simulink model "a_CurrentController_IdealPWMVariousVbusFsw"  (R2013b)
settings: Solver=ode3  StartTime=0.0  StopTime=3e-3  FixedStep=.5e-7  MaxStep=1e-6  RelTol=1e-3
values from neighbouring files (symbols this model uses):
  Ki = R/L*Kp    (= 10000)    [CurrentControllerDesign.m]
  Kp = L*wci    (= 45.2)    [CurrentControllerDesign.m]
  L = 45.2e-3    (= 0.0452)    [CurrentControllerDesign.m]
  R = 10    [CurrentControllerDesign.m]
libraries: fl_lib x28, nesl_utility x14, simulink x6
settings Model: Creator=Eric  LastModifiedBy=sever212
settings DebuggingCC: StateNameClashWarn=warning

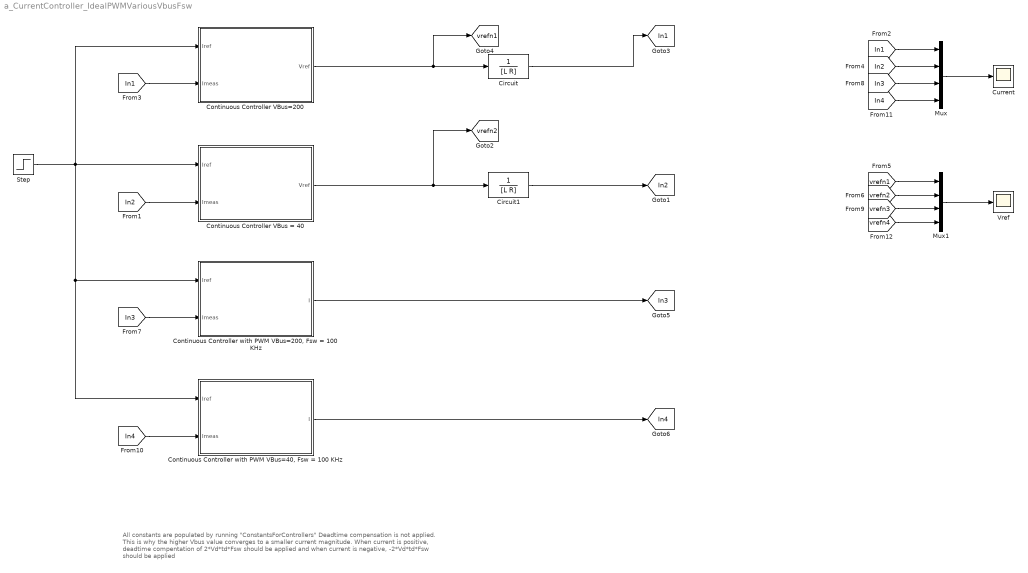
== system a_CurrentController_IdealPWMVariousVbusFsw ==
  note: All constants are populated by running "ConstantsForControllers"
      |
      | Deadtime compensation is not applied. This is why the higher Vbus value converges to a smaller current magnitude.
      |
      | When current is positive, deadtime compentation of 2*Vd*td*Fsw should be applied
      | and when current is negative, -2*Vd*td*Fsw should be applied
  Circuit : TransferFcn  Denominator=[L R]
  Circuit1 : TransferFcn  Denominator=[L R]
  Continuous Controller VBus = 40 : Subsystem  mask{Vdcbus=40}
      mask prompts: Vdcbus "Vdc"
  Continuous Controller VBus=200 : Subsystem  mask{Vdcbus=200}
      mask prompts: Vdcbus "Vdc"
  "Continuous Controller with PWM VBus=200, Fsw = 100 KHz" : Subsystem  mask{Vdcbus=200, fsw=100e3, tdead=80e-9}
      mask prompts: Vdcbus "Vdc"; fsw "Switching Frequency"; tdead "Dead time"
  "Continuous Controller with PWM VBus=40, Fsw = 100 KHz" : Subsystem  mask{Vdcbus=40, fsw=100e3, tdead=80e-9}
      mask prompts: Vdcbus "Vdc"; fsw "Switching Frequency"; tdead "Dead time"
  Current : Scope
      settings: YMin=-1.1  YMax=1.1
  Mux : Mux
  Mux1 : Mux
  Step : Step  Time=1.5e-3  Before=1  After=-1  SampleTime=0
  Vref : Scope
      settings: YMin=-40.5  YMax=-35.5
  tag scope: In1=global, In2=global, In3=global, In4=global, vrefn1=global, vrefn2=global
  wires:
  Continuous Controller VBus=200/1(Vref) -> [vrefn1], Circuit/1
  Circuit/1 -> [In1]
  [In1] -> Continuous Controller VBus=200/2(Imeas)
  [In2] -> Continuous Controller VBus = 40/2(Imeas)
  Continuous Controller VBus = 40/1(Vref) -> [vrefn2], Circuit1/1
  Circuit1/1 -> [In2]
  [In1] -> Mux/1
  [In2] -> Mux/2
  Mux/1 -> Current/1
  [vrefn1] -> Mux1/1
  [vrefn2] -> Mux1/2
  Mux1/1 -> Vref/1
  [In3] -> "Continuous Controller with PWM VBus=200, Fsw = 100 KHz"/2(Imeas)
  "Continuous Controller with PWM VBus=200, Fsw = 100 KHz"/1(I) -> [In3]
  [vrefn3] -> Mux1/3
  [In3] -> Mux/3
  Step/1 -> "Continuous Controller with PWM VBus=200, Fsw = 100 KHz"/1(Iref), "Continuous Controller with PWM VBus=40, Fsw = 100 KHz"/1(Iref), Continuous Controller VBus = 40/1(Iref), Continuous Controller VBus=200/1(Iref)
  [In4] -> "Continuous Controller with PWM VBus=40, Fsw = 100 KHz"/2(Imeas)
  "Continuous Controller with PWM VBus=40, Fsw = 100 KHz"/1(I) -> [In4]
  [In4] -> Mux/4
  [vrefn4] -> Mux1/4

== system a_CurrentController_IdealPWMVariousVbusFsw/Continuous Controller VBus = 40 ==
  Iref : Inport
  Imeas : Inport  Port=2
  Get Error : Subsystem
  PI controller : Subsystem
  Vref : Outport
  wires:
  Get Error/1(Error) -> PI controller/1(error)
  Iref/1 -> Get Error/1(Iref)
  Imeas/1 -> Get Error/2(Imeas)
  PI controller/1(Vref) -> Vref/1

== system a_CurrentController_IdealPWMVariousVbusFsw/Continuous Controller VBus=200 ==
  Iref : Inport
  Imeas : Inport  Port=2
  Get Error : Subsystem
  PI controller : Subsystem
  Vref : Outport
  wires:
  Get Error/1(Error) -> PI controller/1(error)
  Iref/1 -> Get Error/1(Iref)
  Imeas/1 -> Get Error/2(Imeas)
  PI controller/1(Vref) -> Vref/1

== system a_CurrentController_IdealPWMVariousVbusFsw/Continuous Controller with PWM VBus=200, Fsw = 100 KHz ==
  Iref : Inport
  Imeas : Inport  Port=2
  Get Error : Subsystem
  Inverter and Winding2 : Subsystem
  PI controller : Subsystem
  Switching Logic : Subsystem
  Terminator : Terminator
  I : Outport
  tag scope: vrefn3=global
  wires:
  Get Error/1(Error) -> PI controller/1(error)
  Iref/1 -> Get Error/1(Iref)
  Imeas/1 -> Get Error/2(Imeas)
  PI controller/1(Vref) -> [vrefn3], Switching Logic/1(Vref)
  Switching Logic/1(q) -> Inverter and Winding2/1(q)
  Inverter and Winding2/2(V) -> Terminator/1
  Inverter and Winding2/1(I) -> I/1

== system a_CurrentController_IdealPWMVariousVbusFsw/Continuous Controller with PWM VBus=40, Fsw = 100 KHz ==
  Iref : Inport
  Imeas : Inport  Port=2
  Get Error : Subsystem
  Inverter and Winding2 : Subsystem
  PI controller : Subsystem
  Switching Logic : Subsystem
  Terminator : Terminator
  I : Outport
  tag scope: vrefn4=global
  wires:
  Get Error/1(Error) -> PI controller/1(error)
  Iref/1 -> Get Error/1(Iref)
  Imeas/1 -> Get Error/2(Imeas)
  PI controller/1(Vref) -> [vrefn4], Switching Logic/1(Vref)
  Switching Logic/1(q) -> Inverter and Winding2/1(q)
  Inverter and Winding2/2(V) -> Terminator/1
  Inverter and Winding2/1(I) -> I/1

== system a_CurrentController_IdealPWMVariousVbusFsw/Continuous Controller VBus = 40/Get Error ==
  Iref : Inport
  Imeas : Inport  Port=2
  Sum : Sum  Inputs=|+-
  Error : Outport
  wires:
  Sum/1 -> Error/1
  Iref/1 -> Sum/1
  Imeas/1 -> Sum/2

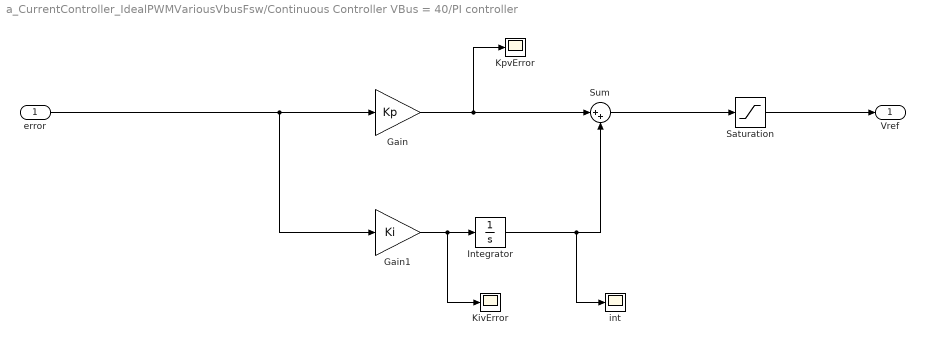
== system a_CurrentController_IdealPWMVariousVbusFsw/Continuous Controller VBus = 40/PI controller ==
  error : Inport
  Gain : Gain  Gain=Kp
  Gain1 : Gain  Gain=Ki
  Integrator : Integrator  LimitOutput=on  UpperSaturationLimit=0.9*Vdcbus  LowerSaturationLimit=-0.9*Vdcbus
  KivError : Scope
      settings: YMin=0.0682  YMax=0.0697  SaveName=ScopeData17
  KpvError : Scope
      settings: YMin=0.0006  YMax=0.00125  SaveName=ScopeData26
  Saturation : Saturate  UpperLimit=0.9*Vdcbus  LowerLimit=-0.9*Vdcbus
  Sum : Sum  Inputs=|++
  int : Scope
      settings: YMin=0.0079765  YMax=0.0079777  SaveName=ScopeData27
  Vref : Outport
  wires:
  error/1 -> Gain1/1, Gain/1
  Gain1/1 -> KivError/1, Integrator/1
  Gain/1 -> KpvError/1, Sum/1
  Integrator/1 -> int/1, Sum/2
  Sum/1 -> Saturation/1
  Saturation/1 -> Vref/1

== system a_CurrentController_IdealPWMVariousVbusFsw/Continuous Controller VBus=200/Get Error ==
  Iref : Inport
  Imeas : Inport  Port=2
  Sum : Sum  Inputs=|+-
  Error : Outport
  wires:
  Sum/1 -> Error/1
  Iref/1 -> Sum/1
  Imeas/1 -> Sum/2

== system a_CurrentController_IdealPWMVariousVbusFsw/Continuous Controller VBus=200/PI controller ==
  error : Inport
  Gain : Gain  Gain=Kp
  Gain1 : Gain  Gain=Ki
  Integrator : Integrator  LimitOutput=on  UpperSaturationLimit=0.9*Vdcbus  LowerSaturationLimit=-0.9*Vdcbus
  KivError : Scope
      settings: YMin=0.0682  YMax=0.0697  SaveName=ScopeData17
  KpvError : Scope
      settings: YMin=0.0006  YMax=0.00125  SaveName=ScopeData26
  Saturation : Saturate  UpperLimit=0.9*Vdcbus  LowerLimit=-0.9*Vdcbus
  Sum : Sum  Inputs=|++
  int : Scope
      settings: YMin=0.0079765  YMax=0.0079777  SaveName=ScopeData27
  Vref : Outport
  wires:
  error/1 -> Gain1/1, Gain/1
  Gain1/1 -> KivError/1, Integrator/1
  Gain/1 -> KpvError/1, Sum/1
  Integrator/1 -> int/1, Sum/2
  Sum/1 -> Saturation/1
  Saturation/1 -> Vref/1

== system a_CurrentController_IdealPWMVariousVbusFsw/Continuous Controller with PWM VBus=200, Fsw = 100 KHz/Get Error ==
  Iref : Inport
  Imeas : Inport  Port=2
  Sum : Sum  Inputs=|+-
  Error : Outport
  wires:
  Sum/1 -> Error/1
  Iref/1 -> Sum/1
  Imeas/1 -> Sum/2

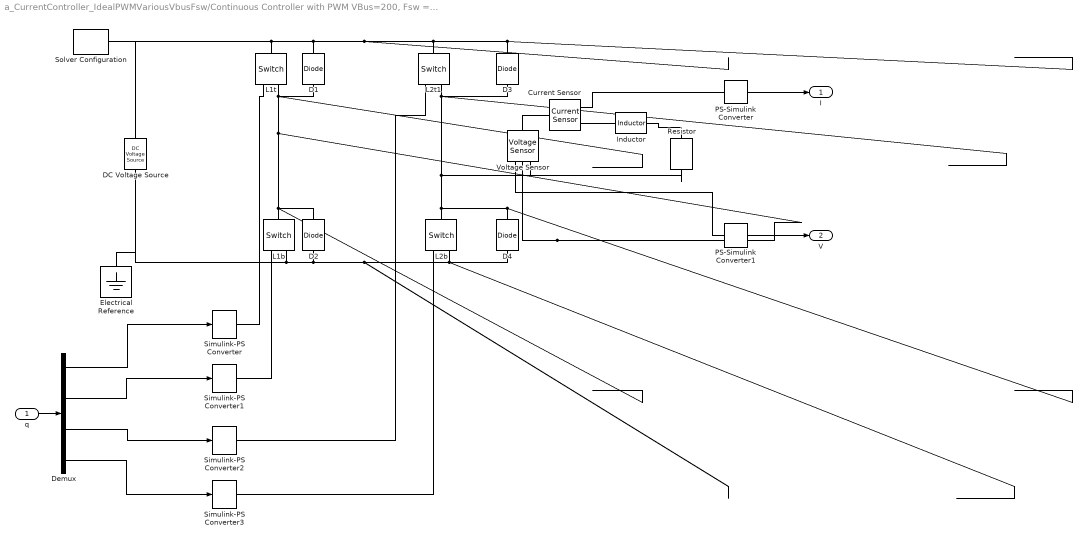
== system a_CurrentController_IdealPWMVariousVbusFsw/Continuous Controller with PWM VBus=200, Fsw = 100 KHz/Inverter and Winding2 ==
  q : Inport
  Current Sensor : fl_lib/Electrical/Electrical Sensors/Current Sensor  i1_Log=off  v1_Log=off  LocalVarNames=|i1|v1  LocalVarDescs=|i1|v1  LocalVarLogging=[0 0]
  D{1..4} (4 alike) : fl_lib/Electrical/Electrical Elements/Diode  Vf=0.15 V  Ron=0.01 Ohm  Goff=1e-7 1/Ohm  i_Log=off  v_Log=off  LocalVarNames=|i|v  LocalVarDescs=|i|v  LocalVarLogging=[0 0]
  DC Voltage Source : fl_lib/Electrical/Electrical Sources/DC Voltage Source  v0=Vdcbus V  i_Log=off  v_Log=off  LocalVarNames=|i|v  LocalVarDescs=|i|v  LocalVarLogging=[0 0]
  Demux : Demux
  Electrical Reference : fl_lib/Electrical/Electrical Elements/Electrical Reference  i_Log=off  LocalVarNames=|i  LocalVarDescs=|i  LocalVarLogging=0
  Inductor : fl_lib/Electrical/Electrical Elements/Inductor  l=L H  i0=0 A  r=0 Ohm  g=1e-8 1/Ohm  i_Log=off  v_Log=off  i_L_Log=off  LocalVarNames=|i|v|i_L  LocalVarDescs=|i|v|Internal variable for current through inductor term  LocalVarLogging=[0 0 0]
  L1b : fl_lib/Electrical/Electrical Elements/Switch  R_closed=0.01 Ohm  G_open=1e-7 1/Ohm  Threshold=0.1  i_Log=off  v_Log=off  LocalVarNames=|i|v  LocalVarDescs=|i|v  LocalVarLogging=[0 0]
  L1t : fl_lib/Electrical/Electrical Elements/Switch  R_closed=0.01 Ohm  G_open=1e-7 1/Ohm  Threshold=0.1  i_Log=off  v_Log=off  LocalVarNames=|i|v  LocalVarDescs=|i|v  LocalVarLogging=[0 0]
  L2b : fl_lib/Electrical/Electrical Elements/Switch  R_closed=0.01 Ohm  G_open=1e-7 1/Ohm  Threshold=0.1  i_Log=off  v_Log=off  LocalVarNames=|i|v  LocalVarDescs=|i|v  LocalVarLogging=[0 0]
  L2t1 : fl_lib/Electrical/Electrical Elements/Switch  R_closed=0.01 Ohm  G_open=1e-7 1/Ohm  Threshold=0.1  i_Log=off  v_Log=off  LocalVarNames=|i|v  LocalVarDescs=|i|v  LocalVarLogging=[0 0]
  PS-Simulink Converter : nesl_utility/PS-Simulink Converter  PhysicalDomain=network_engine_domain  SubClassName=ps_output  LeftPortType=input  RightPortType=output  PseudoPeriodic=off  Frequencies=[]  Unit=1  AffineConversion=off
  PS-Simulink Converter1 : nesl_utility/PS-Simulink Converter  PhysicalDomain=network_engine_domain  SubClassName=ps_output  LeftPortType=input  RightPortType=output  PseudoPeriodic=off  Frequencies=[]  Unit=1  AffineConversion=off
  Resistor : fl_lib/Electrical/Electrical Elements/Resistor  R=R Ohm  i_Log=off  v_Log=off  LocalVarNames=|i|v  LocalVarDescs=|i|v  LocalVarLogging=[0 0]
  Simulink-PS Converter{,1..3} (4 alike) : nesl_utility/Simulink-PS Converter  PhysicalDomain=network_engine_domain  SubClassName=ps_input  LeftPortType=input  RightPortType=output  PseudoPeriodic=off  Frequencies=[]  NoiseDistribution=none  NoiseParameters=[]  Unit=1  AffineConversion=off  InputFiltering=off  SimscapeFilterOrder=1  InputFilterTimeConstant=.001  UdotUserProvided=[]
  Solver Configuration : nesl_utility/Solver Configuration  PhysicalDomain=network_engine_domain  SubClassName=solver  LeftPortType=input  RightPortType=generic  Accelerate=off  Tones=[]  Harmonics=[]  SimulateNoise=off  Profile=off  UseLocalSampling=off  EnableSwitchedLinearOptims=on  FrequencyDomain=off  UseCCode=off  RelTol=0.001  AbsTol=1e-06  MinStep=1e-09  ToWorkspace=off  DoDC=on  ResidualTolerance=1e-8  UseLocalSolver=off  LocalSolverChoice=NE_BACKWARD_EULER_ADVANCER  LocalSolverSampleTime=100e-9  DoFixedCost=off  MaxNonlinIter=15  MaxModeIter=2  LinearAlgebra=Sparse  DelaysMemoryBudget=1024
  Voltage Sensor : fl_lib/Electrical/Electrical Sensors/Voltage Sensor  i1_Log=off  v1_Log=off  LocalVarNames=|i1|v1  LocalVarDescs=|i1|v1  LocalVarLogging=[0 0]
  I : Outport
  V : Outport  Port=2
  wires:
  PS-Simulink Converter/1 -> I/1
  PS-Simulink Converter1/1 -> V/1
  q/1 -> Demux/1
  Demux/1 -> Simulink-PS Converter/1
  Demux/2 -> Simulink-PS Converter1/1
  Demux/3 -> Simulink-PS Converter2/1
  Demux/4 -> Simulink-PS Converter3/1
  connections:
  L1t/RConn2 -- D1/LConn1 -- Voltage Sensor/LConn1 -- Current Sensor/LConn1 -- D2/RConn1 -- L1b/LConn1
  Inductor/RConn1 -- Resistor/LConn1
  Simulink-PS Converter2/RConn1 -- L2t1/RConn1
  Simulink-PS Converter/RConn1 -- L1t/RConn1
  Simulink-PS Converter1/RConn1 -- L1b/RConn1
  D4/RConn1 -- Voltage Sensor/RConn2 -- Resistor/RConn1 -- D3/LConn1 -- L2t1/RConn2 -- L2b/LConn1
  L1b/RConn2 -- Electrical Reference/LConn1 -- DC Voltage Source/RConn1 -- D2/LConn1 -- D4/LConn1 -- L2b/RConn2
  L1t/LConn1 -- L2t1/LConn1 -- D3/RConn1 -- D1/RConn1 -- Solver Configuration/RConn1 -- DC Voltage Source/LConn1
  Simulink-PS Converter3/RConn1 -- L2b/RConn1
  Current Sensor/RConn2 -- Inductor/LConn1
  Current Sensor/RConn1 -- PS-Simulink Converter/LConn1
  Voltage Sensor/RConn1 -- PS-Simulink Converter1/LConn1

== system a_CurrentController_IdealPWMVariousVbusFsw/Continuous Controller with PWM VBus=200, Fsw = 100 KHz/PI controller ==
  error : Inport
  Gain : Gain  Gain=Kp
  Gain1 : Gain  Gain=Ki
  Integrator : Integrator  LimitOutput=on  UpperSaturationLimit=0.9*Vdcbus  LowerSaturationLimit=-0.9*Vdcbus
  KivError : Scope
      settings: YMin=0.0682  YMax=0.0697  SaveName=ScopeData17
  KpvError : Scope
      settings: YMin=0.0006  YMax=0.00125  SaveName=ScopeData26
  Saturation : Saturate  UpperLimit=0.9*Vdcbus  LowerLimit=-0.9*Vdcbus
  Sum : Sum  Inputs=|++
  int : Scope
      settings: YMin=0.0079765  YMax=0.0079777  SaveName=ScopeData27
  Vref : Outport
  wires:
  error/1 -> Gain1/1, Gain/1
  Gain1/1 -> KivError/1, Integrator/1
  Gain/1 -> KpvError/1, Sum/1
  Integrator/1 -> int/1, Sum/2
  Sum/1 -> Saturation/1
  Saturation/1 -> Vref/1

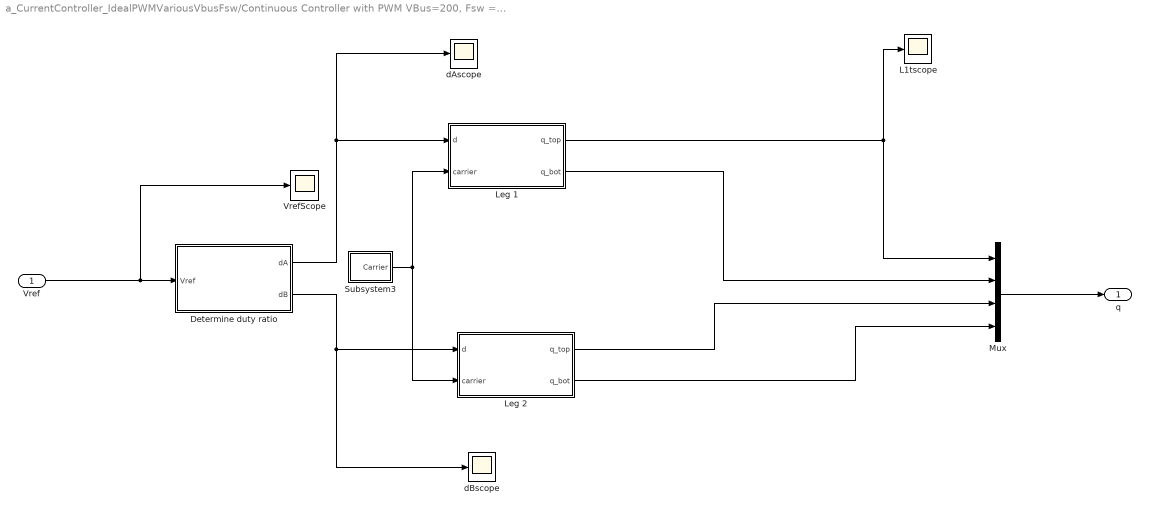
== system a_CurrentController_IdealPWMVariousVbusFsw/Continuous Controller with PWM VBus=200, Fsw = 100 KHz/Switching Logic ==
  Vref : Inport
  Determine duty ratio : Subsystem
  L1tscope : Scope
  Leg 1 : Subsystem
  Leg 2 : Subsystem
  Mux : Mux
  Subsystem3 : Subsystem
  VrefScope : Scope
      settings: YMin=-0.076  YMax=-0.074  SaveName=ScopeData4
  dAscope : Scope
      settings: YMin=0.462  YMax=0.463  SaveName=ScopeData6
  dBscope : Scope
      settings: SaveName=ScopeData7
  q : Outport
  wires:
  Subsystem3/1(Carrier) -> Leg 2/2(carrier), Leg 1/2(carrier)
  Determine duty ratio/2(dB) -> Leg 2/1(d), dBscope/1
  Determine duty ratio/1(dA) -> Leg 1/1(d), dAscope/1
  Vref/1 -> VrefScope/1, Determine duty ratio/1(Vref)
  Leg 1/1(q_top) -> Mux/1, L1tscope/1
  Leg 2/1(q_top) -> Mux/3
  Leg 2/2(q_bot) -> Mux/4
  Mux/1 -> q/1
  Leg 1/2(q_bot) -> Mux/2

== system a_CurrentController_IdealPWMVariousVbusFsw/Continuous Controller with PWM VBus=40, Fsw = 100 KHz/Get Error ==
  Iref : Inport
  Imeas : Inport  Port=2
  Sum : Sum  Inputs=|+-
  Error : Outport
  wires:
  Sum/1 -> Error/1
  Iref/1 -> Sum/1
  Imeas/1 -> Sum/2

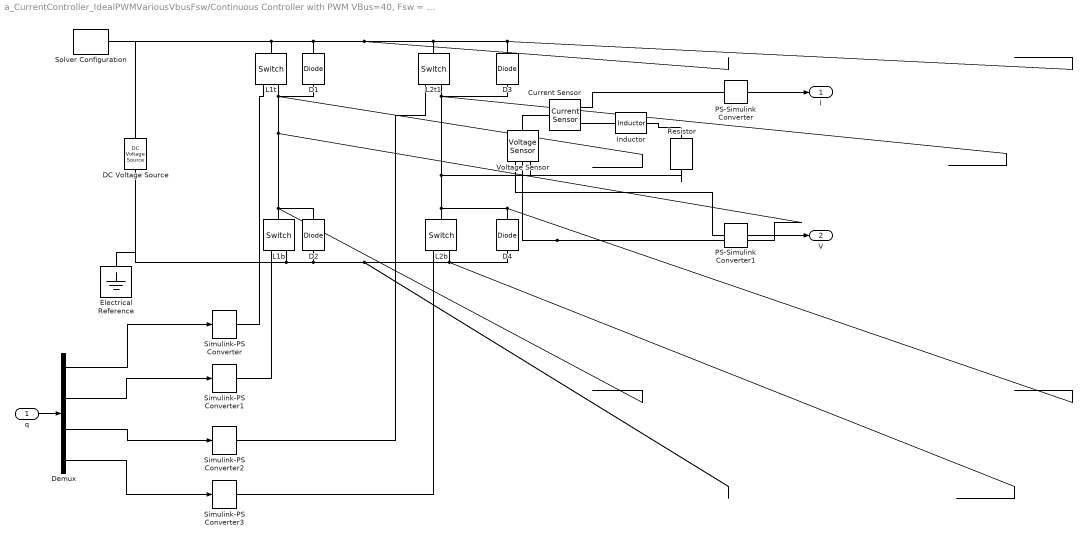
== system a_CurrentController_IdealPWMVariousVbusFsw/Continuous Controller with PWM VBus=40, Fsw = 100 KHz/Inverter and Winding2 ==
  q : Inport
  Current Sensor : fl_lib/Electrical/Electrical Sensors/Current Sensor  i1_Log=off  v1_Log=off  LocalVarNames=|i1|v1  LocalVarDescs=|i1|v1  LocalVarLogging=[0 0]
  D{1..4} (4 alike) : fl_lib/Electrical/Electrical Elements/Diode  Vf=0.15 V  Ron=0.01 Ohm  Goff=1e-7 1/Ohm  i_Log=off  v_Log=off  LocalVarNames=|i|v  LocalVarDescs=|i|v  LocalVarLogging=[0 0]
  DC Voltage Source : fl_lib/Electrical/Electrical Sources/DC Voltage Source  v0=Vdcbus V  i_Log=off  v_Log=off  LocalVarNames=|i|v  LocalVarDescs=|i|v  LocalVarLogging=[0 0]
  Demux : Demux
  Electrical Reference : fl_lib/Electrical/Electrical Elements/Electrical Reference  i_Log=off  LocalVarNames=|i  LocalVarDescs=|i  LocalVarLogging=0
  Inductor : fl_lib/Electrical/Electrical Elements/Inductor  l=L H  i0=0 A  r=0 Ohm  g=1e-8 1/Ohm  i_Log=off  v_Log=off  i_L_Log=off  LocalVarNames=|i|v|i_L  LocalVarDescs=|i|v|Internal variable for current through inductor term  LocalVarLogging=[0 0 0]
  L1b : fl_lib/Electrical/Electrical Elements/Switch  R_closed=0.01 Ohm  G_open=1e-7 1/Ohm  Threshold=0.1  i_Log=off  v_Log=off  LocalVarNames=|i|v  LocalVarDescs=|i|v  LocalVarLogging=[0 0]
  L1t : fl_lib/Electrical/Electrical Elements/Switch  R_closed=0.01 Ohm  G_open=1e-7 1/Ohm  Threshold=0.1  i_Log=off  v_Log=off  LocalVarNames=|i|v  LocalVarDescs=|i|v  LocalVarLogging=[0 0]
  L2b : fl_lib/Electrical/Electrical Elements/Switch  R_closed=0.01 Ohm  G_open=1e-7 1/Ohm  Threshold=0.1  i_Log=off  v_Log=off  LocalVarNames=|i|v  LocalVarDescs=|i|v  LocalVarLogging=[0 0]
  L2t1 : fl_lib/Electrical/Electrical Elements/Switch  R_closed=0.01 Ohm  G_open=1e-7 1/Ohm  Threshold=0.1  i_Log=off  v_Log=off  LocalVarNames=|i|v  LocalVarDescs=|i|v  LocalVarLogging=[0 0]
  PS-Simulink Converter : nesl_utility/PS-Simulink Converter  PhysicalDomain=network_engine_domain  SubClassName=ps_output  LeftPortType=input  RightPortType=output  PseudoPeriodic=off  Frequencies=[]  Unit=1  AffineConversion=off
  PS-Simulink Converter1 : nesl_utility/PS-Simulink Converter  PhysicalDomain=network_engine_domain  SubClassName=ps_output  LeftPortType=input  RightPortType=output  PseudoPeriodic=off  Frequencies=[]  Unit=1  AffineConversion=off
  Resistor : fl_lib/Electrical/Electrical Elements/Resistor  R=R Ohm  i_Log=off  v_Log=off  LocalVarNames=|i|v  LocalVarDescs=|i|v  LocalVarLogging=[0 0]
  Simulink-PS Converter{,1..3} (4 alike) : nesl_utility/Simulink-PS Converter  PhysicalDomain=network_engine_domain  SubClassName=ps_input  LeftPortType=input  RightPortType=output  PseudoPeriodic=off  Frequencies=[]  NoiseDistribution=none  NoiseParameters=[]  Unit=1  AffineConversion=off  InputFiltering=off  SimscapeFilterOrder=1  InputFilterTimeConstant=.001  UdotUserProvided=[]
  Solver Configuration : nesl_utility/Solver Configuration  PhysicalDomain=network_engine_domain  SubClassName=solver  LeftPortType=input  RightPortType=generic  Accelerate=off  Tones=[]  Harmonics=[]  SimulateNoise=off  Profile=off  UseLocalSampling=off  EnableSwitchedLinearOptims=on  FrequencyDomain=off  UseCCode=off  RelTol=0.001  AbsTol=1e-06  MinStep=1e-09  ToWorkspace=off  DoDC=on  ResidualTolerance=1e-8  UseLocalSolver=off  LocalSolverChoice=NE_BACKWARD_EULER_ADVANCER  LocalSolverSampleTime=100e-9  DoFixedCost=off  MaxNonlinIter=15  MaxModeIter=2  LinearAlgebra=Sparse  DelaysMemoryBudget=1024
  Voltage Sensor : fl_lib/Electrical/Electrical Sensors/Voltage Sensor  i1_Log=off  v1_Log=off  LocalVarNames=|i1|v1  LocalVarDescs=|i1|v1  LocalVarLogging=[0 0]
  I : Outport
  V : Outport  Port=2
  wires:
  PS-Simulink Converter/1 -> I/1
  PS-Simulink Converter1/1 -> V/1
  q/1 -> Demux/1
  Demux/1 -> Simulink-PS Converter/1
  Demux/2 -> Simulink-PS Converter1/1
  Demux/3 -> Simulink-PS Converter2/1
  Demux/4 -> Simulink-PS Converter3/1
  connections:
  L1t/RConn2 -- D1/LConn1 -- Voltage Sensor/LConn1 -- Current Sensor/LConn1 -- D2/RConn1 -- L1b/LConn1
  Inductor/RConn1 -- Resistor/LConn1
  Simulink-PS Converter2/RConn1 -- L2t1/RConn1
  Simulink-PS Converter/RConn1 -- L1t/RConn1
  Simulink-PS Converter1/RConn1 -- L1b/RConn1
  D4/RConn1 -- Voltage Sensor/RConn2 -- Resistor/RConn1 -- D3/LConn1 -- L2t1/RConn2 -- L2b/LConn1
  L1b/RConn2 -- Electrical Reference/LConn1 -- DC Voltage Source/RConn1 -- D2/LConn1 -- D4/LConn1 -- L2b/RConn2
  L1t/LConn1 -- L2t1/LConn1 -- D3/RConn1 -- D1/RConn1 -- Solver Configuration/RConn1 -- DC Voltage Source/LConn1
  Simulink-PS Converter3/RConn1 -- L2b/RConn1
  Current Sensor/RConn2 -- Inductor/LConn1
  Current Sensor/RConn1 -- PS-Simulink Converter/LConn1
  Voltage Sensor/RConn1 -- PS-Simulink Converter1/LConn1

== system a_CurrentController_IdealPWMVariousVbusFsw/Continuous Controller with PWM VBus=40, Fsw = 100 KHz/PI controller ==
  error : Inport
  Gain : Gain  Gain=Kp
  Gain1 : Gain  Gain=Ki
  Integrator : Integrator  LimitOutput=on  UpperSaturationLimit=0.9*Vdcbus  LowerSaturationLimit=-0.9*Vdcbus
  KivError : Scope
      settings: YMin=0.0682  YMax=0.0697  SaveName=ScopeData17
  KpvError : Scope
      settings: YMin=0.0006  YMax=0.00125  SaveName=ScopeData26
  Saturation : Saturate  UpperLimit=0.9*Vdcbus  LowerLimit=-0.9*Vdcbus
  Sum : Sum  Inputs=|++
  int : Scope
      settings: YMin=0.0079765  YMax=0.0079777  SaveName=ScopeData27
  Vref : Outport
  wires:
  error/1 -> Gain1/1, Gain/1
  Gain1/1 -> KivError/1, Integrator/1
  Gain/1 -> KpvError/1, Sum/1
  Integrator/1 -> int/1, Sum/2
  Sum/1 -> Saturation/1
  Saturation/1 -> Vref/1

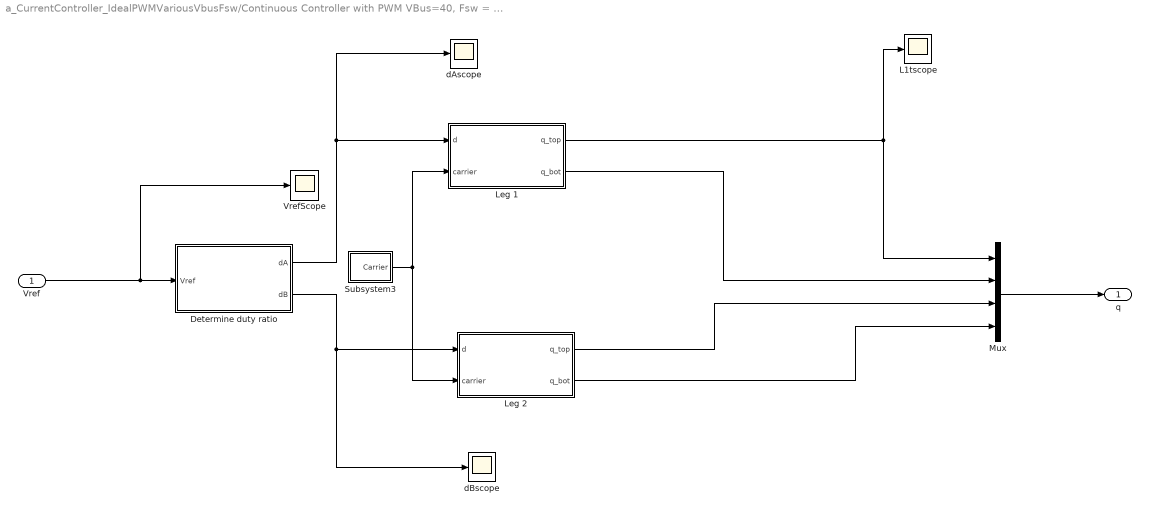
== system a_CurrentController_IdealPWMVariousVbusFsw/Continuous Controller with PWM VBus=40, Fsw = 100 KHz/Switching Logic ==
  Vref : Inport
  Determine duty ratio : Subsystem
  L1tscope : Scope
  Leg 1 : Subsystem
  Leg 2 : Subsystem
  Mux : Mux
  Subsystem3 : Subsystem
  VrefScope : Scope
      settings: YMin=-0.076  YMax=-0.074  SaveName=ScopeData4
  dAscope : Scope
      settings: YMin=0.462  YMax=0.463  SaveName=ScopeData6
  dBscope : Scope
      settings: SaveName=ScopeData7
  q : Outport
  wires:
  Subsystem3/1(Carrier) -> Leg 2/2(carrier), Leg 1/2(carrier)
  Determine duty ratio/2(dB) -> Leg 2/1(d), dBscope/1
  Determine duty ratio/1(dA) -> Leg 1/1(d), dAscope/1
  Vref/1 -> VrefScope/1, Determine duty ratio/1(Vref)
  Leg 1/1(q_top) -> Mux/1, L1tscope/1
  Leg 2/1(q_top) -> Mux/3
  Leg 2/2(q_bot) -> Mux/4
  Mux/1 -> q/1
  Leg 1/2(q_bot) -> Mux/2

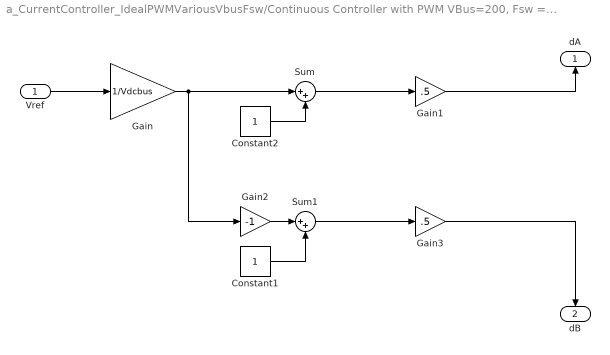
== system a_CurrentController_IdealPWMVariousVbusFsw/Continuous Controller with PWM VBus=200, Fsw = 100 KHz/Switching Logic/Determine duty ratio ==
  Vref : Inport
  Constant1 : Constant
  Constant2 : Constant
  Gain : Gain  Gain=1/Vdcbus
  Gain1 : Gain  Gain=.5
  Gain2 : Gain  Gain=-1
  Gain3 : Gain  Gain=.5
  Sum : Sum  Inputs=|++
  Sum1 : Sum  Inputs=|++
  dA : Outport
  dB : Outport  Port=2
  wires:
  Vref/1 -> Gain/1
  Gain/1 -> Gain2/1, Sum/1
  Sum/1 -> Gain1/1
  Gain2/1 -> Sum1/1
  Gain1/1 -> dA/1
  Constant2/1 -> Sum/2
  Constant1/1 -> Sum1/2
  Sum1/1 -> Gain3/1
  Gain3/1 -> dB/1

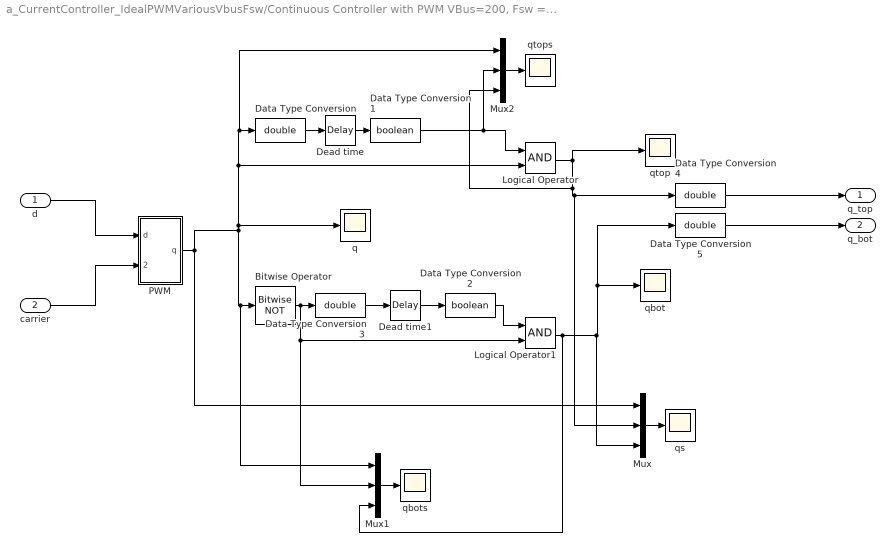
== system a_CurrentController_IdealPWMVariousVbusFsw/Continuous Controller with PWM VBus=200, Fsw = 100 KHz/Switching Logic/Leg 1 ==
  d : Inport
  carrier : Inport  Port=2
  Bitwise Operator : simulink/Logic and Bit Operations/Bitwise Operator  logicop=NOT  UseBitMask=off  BitMask=bin2dec('11011001')  BitMaskRealWorld=Stored Integer
  Data Type Conversion{,3..5} (4 alike) : DataTypeConversion  OutDataTypeStr=double
  Data Type Conversion1 : DataTypeConversion  OutDataTypeStr=boolean
  Data Type Conversion2 : DataTypeConversion  OutDataTypeStr=boolean
  Dead time : TransportDelay  DelayTime=tdead
  Dead time1 : TransportDelay  DelayTime=tdead
  Logical Operator : Logic  AllPortsSameDT=off  OutDataTypeStr=boolean
  Logical Operator1 : Logic  AllPortsSameDT=off  OutDataTypeStr=boolean
  Mux : Mux  Inputs=3
  Mux1 : Mux  Inputs=3
  Mux2 : Mux  Inputs=3
  PWM : Subsystem
  q : Scope
      settings: SaveName=ScopeData5
  qbot : Scope
      settings: SaveName=ScopeData8
  qbots : Scope
      settings: SaveName=ScopeData11
  qs : Scope
      settings: SaveName=ScopeData10
  qtop : Scope
      settings: SaveName=ScopeData9
  qtops : Scope
      settings: YMin=-0.1  YMax=2  SaveName=ScopeData12
  q_top : Outport
  q_bot : Outport  Port=2
  wires:
  d/1 -> PWM/1(d)
  PWM/1(q) -> Mux/1, Mux1/1, Bitwise Operator/1, q/1, Mux2/1, Data Type Conversion/1, Logical Operator/2
  Logical Operator/1 -> Mux2/3, Mux/2, Data Type Conversion4/1, qtop/1
  carrier/1 -> PWM/2(carrier)
  Dead time/1 -> Data Type Conversion1/1
  Bitwise Operator/1 -> Logical Operator1/2, Mux1/2, Data Type Conversion3/1
  Dead time1/1 -> Data Type Conversion2/1
  Logical Operator1/1 -> Mux1/3, Mux/3, qbot/1, Data Type Conversion5/1
  Data Type Conversion1/1 -> Mux2/2, Logical Operator/1
  Data Type Conversion/1 -> Dead time/1
  Data Type Conversion2/1 -> Logical Operator1/1
  Data Type Conversion3/1 -> Dead time1/1
  Mux/1 -> qs/1
  Mux1/1 -> qbots/1
  Mux2/1 -> qtops/1
  Data Type Conversion4/1 -> q_top/1
  Data Type Conversion5/1 -> q_bot/1

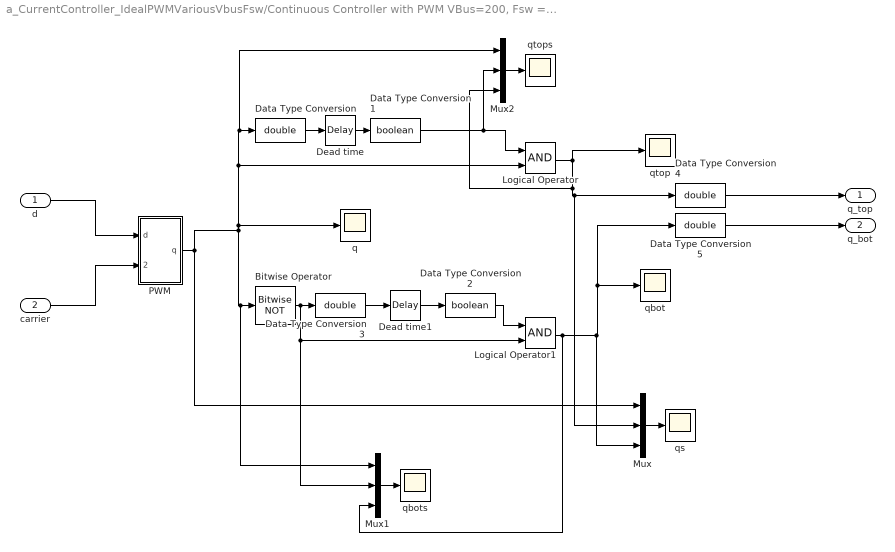
== system a_CurrentController_IdealPWMVariousVbusFsw/Continuous Controller with PWM VBus=200, Fsw = 100 KHz/Switching Logic/Leg 2 ==
  d : Inport
  carrier : Inport  Port=2
  Bitwise Operator : simulink/Logic and Bit Operations/Bitwise Operator  logicop=NOT  UseBitMask=off  BitMask=bin2dec('11011001')  BitMaskRealWorld=Stored Integer
  Data Type Conversion{,3..5} (4 alike) : DataTypeConversion  OutDataTypeStr=double
  Data Type Conversion1 : DataTypeConversion  OutDataTypeStr=boolean
  Data Type Conversion2 : DataTypeConversion  OutDataTypeStr=boolean
  Dead time : TransportDelay  DelayTime=tdead
  Dead time1 : TransportDelay  DelayTime=tdead
  Logical Operator : Logic  AllPortsSameDT=off  OutDataTypeStr=boolean
  Logical Operator1 : Logic  AllPortsSameDT=off  OutDataTypeStr=boolean
  Mux : Mux  Inputs=3
  Mux1 : Mux  Inputs=3
  Mux2 : Mux  Inputs=3
  PWM : Subsystem
  q : Scope
      settings: SaveName=ScopeData5
  qbot : Scope
      settings: SaveName=ScopeData8
  qbots : Scope
      settings: SaveName=ScopeData11
  qs : Scope
      settings: SaveName=ScopeData10
  qtop : Scope
      settings: SaveName=ScopeData9
  qtops : Scope
      settings: YMin=-0.1  YMax=2  SaveName=ScopeData12
  q_top : Outport
  q_bot : Outport  Port=2
  wires:
  d/1 -> PWM/1(d)
  PWM/1(q) -> Mux/1, Mux1/1, Bitwise Operator/1, q/1, Mux2/1, Data Type Conversion/1, Logical Operator/2
  Logical Operator/1 -> Mux2/3, Mux/2, Data Type Conversion4/1, qtop/1
  carrier/1 -> PWM/2(carrier)
  Dead time/1 -> Data Type Conversion1/1
  Bitwise Operator/1 -> Logical Operator1/2, Mux1/2, Data Type Conversion3/1
  Dead time1/1 -> Data Type Conversion2/1
  Logical Operator1/1 -> Mux1/3, Mux/3, qbot/1, Data Type Conversion5/1
  Data Type Conversion1/1 -> Mux2/2, Logical Operator/1
  Data Type Conversion/1 -> Dead time/1
  Data Type Conversion2/1 -> Logical Operator1/1
  Data Type Conversion3/1 -> Dead time1/1
  Mux/1 -> qs/1
  Mux1/1 -> qbots/1
  Mux2/1 -> qtops/1
  Data Type Conversion4/1 -> q_top/1
  Data Type Conversion5/1 -> q_bot/1

== system a_CurrentController_IdealPWMVariousVbusFsw/Continuous Controller with PWM VBus=200, Fsw = 100 KHz/Switching Logic/Subsystem3 ==
  Carrier signal : simulink/Sources/Repeating Sequence  rep_seq_t=[0 .5 1]/fsw  rep_seq_y=[0 1 0]
  Scope : Scope
      settings: SaveName=ScopeData3
  Carrier : Outport
  wires:
  Carrier signal/1 -> Scope/1, Carrier/1

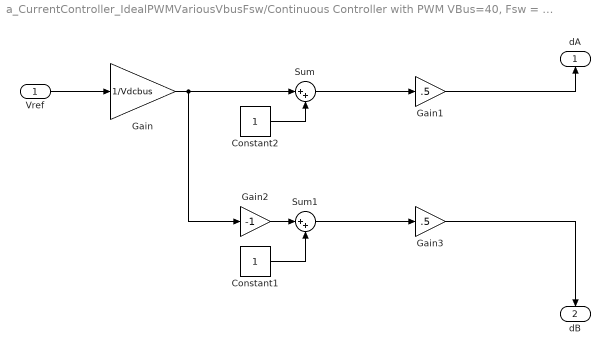
== system a_CurrentController_IdealPWMVariousVbusFsw/Continuous Controller with PWM VBus=40, Fsw = 100 KHz/Switching Logic/Determine duty ratio ==
  Vref : Inport
  Constant1 : Constant
  Constant2 : Constant
  Gain : Gain  Gain=1/Vdcbus
  Gain1 : Gain  Gain=.5
  Gain2 : Gain  Gain=-1
  Gain3 : Gain  Gain=.5
  Sum : Sum  Inputs=|++
  Sum1 : Sum  Inputs=|++
  dA : Outport
  dB : Outport  Port=2
  wires:
  Vref/1 -> Gain/1
  Gain/1 -> Gain2/1, Sum/1
  Sum/1 -> Gain1/1
  Gain2/1 -> Sum1/1
  Gain1/1 -> dA/1
  Constant2/1 -> Sum/2
  Constant1/1 -> Sum1/2
  Sum1/1 -> Gain3/1
  Gain3/1 -> dB/1

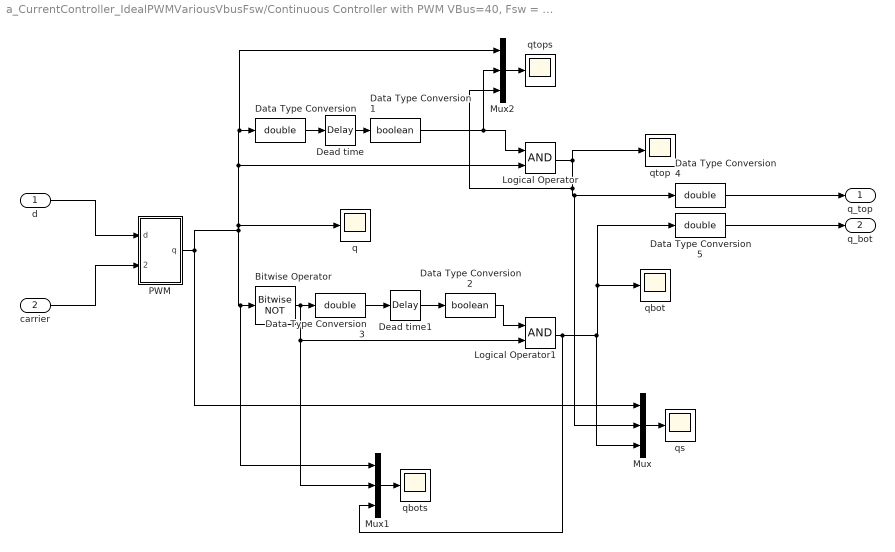
== system a_CurrentController_IdealPWMVariousVbusFsw/Continuous Controller with PWM VBus=40, Fsw = 100 KHz/Switching Logic/Leg 1 ==
  d : Inport
  carrier : Inport  Port=2
  Bitwise Operator : simulink/Logic and Bit Operations/Bitwise Operator  logicop=NOT  UseBitMask=off  BitMask=bin2dec('11011001')  BitMaskRealWorld=Stored Integer
  Data Type Conversion{,3..5} (4 alike) : DataTypeConversion  OutDataTypeStr=double
  Data Type Conversion1 : DataTypeConversion  OutDataTypeStr=boolean
  Data Type Conversion2 : DataTypeConversion  OutDataTypeStr=boolean
  Dead time : TransportDelay  DelayTime=tdead
  Dead time1 : TransportDelay  DelayTime=tdead
  Logical Operator : Logic  AllPortsSameDT=off  OutDataTypeStr=boolean
  Logical Operator1 : Logic  AllPortsSameDT=off  OutDataTypeStr=boolean
  Mux : Mux  Inputs=3
  Mux1 : Mux  Inputs=3
  Mux2 : Mux  Inputs=3
  PWM : Subsystem
  q : Scope
      settings: SaveName=ScopeData5
  qbot : Scope
      settings: SaveName=ScopeData8
  qbots : Scope
      settings: SaveName=ScopeData11
  qs : Scope
      settings: SaveName=ScopeData10
  qtop : Scope
      settings: SaveName=ScopeData9
  qtops : Scope
      settings: YMin=-0.1  YMax=2  SaveName=ScopeData12
  q_top : Outport
  q_bot : Outport  Port=2
  wires:
  d/1 -> PWM/1(d)
  PWM/1(q) -> Mux/1, Mux1/1, Bitwise Operator/1, q/1, Mux2/1, Data Type Conversion/1, Logical Operator/2
  Logical Operator/1 -> Mux2/3, Mux/2, Data Type Conversion4/1, qtop/1
  carrier/1 -> PWM/2(carrier)
  Dead time/1 -> Data Type Conversion1/1
  Bitwise Operator/1 -> Logical Operator1/2, Mux1/2, Data Type Conversion3/1
  Dead time1/1 -> Data Type Conversion2/1
  Logical Operator1/1 -> Mux1/3, Mux/3, qbot/1, Data Type Conversion5/1
  Data Type Conversion1/1 -> Mux2/2, Logical Operator/1
  Data Type Conversion/1 -> Dead time/1
  Data Type Conversion2/1 -> Logical Operator1/1
  Data Type Conversion3/1 -> Dead time1/1
  Mux/1 -> qs/1
  Mux1/1 -> qbots/1
  Mux2/1 -> qtops/1
  Data Type Conversion4/1 -> q_top/1
  Data Type Conversion5/1 -> q_bot/1

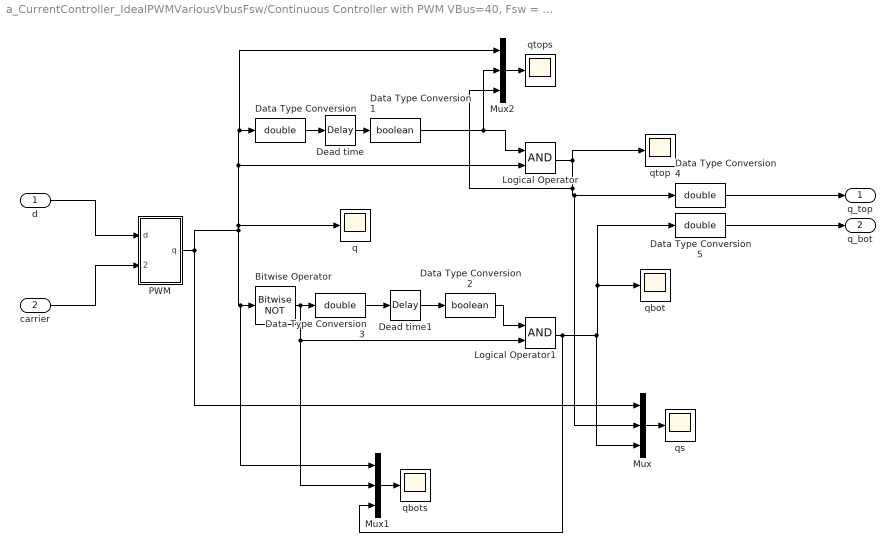
== system a_CurrentController_IdealPWMVariousVbusFsw/Continuous Controller with PWM VBus=40, Fsw = 100 KHz/Switching Logic/Leg 2 ==
  d : Inport
  carrier : Inport  Port=2
  Bitwise Operator : simulink/Logic and Bit Operations/Bitwise Operator  logicop=NOT  UseBitMask=off  BitMask=bin2dec('11011001')  BitMaskRealWorld=Stored Integer
  Data Type Conversion{,3..5} (4 alike) : DataTypeConversion  OutDataTypeStr=double
  Data Type Conversion1 : DataTypeConversion  OutDataTypeStr=boolean
  Data Type Conversion2 : DataTypeConversion  OutDataTypeStr=boolean
  Dead time : TransportDelay  DelayTime=tdead
  Dead time1 : TransportDelay  DelayTime=tdead
  Logical Operator : Logic  AllPortsSameDT=off  OutDataTypeStr=boolean
  Logical Operator1 : Logic  AllPortsSameDT=off  OutDataTypeStr=boolean
  Mux : Mux  Inputs=3
  Mux1 : Mux  Inputs=3
  Mux2 : Mux  Inputs=3
  PWM : Subsystem
  q : Scope
      settings: SaveName=ScopeData5
  qbot : Scope
      settings: SaveName=ScopeData8
  qbots : Scope
      settings: SaveName=ScopeData11
  qs : Scope
      settings: SaveName=ScopeData10
  qtop : Scope
      settings: SaveName=ScopeData9
  qtops : Scope
      settings: YMin=-0.1  YMax=2  SaveName=ScopeData12
  q_top : Outport
  q_bot : Outport  Port=2
  wires:
  d/1 -> PWM/1(d)
  PWM/1(q) -> Mux/1, Mux1/1, Bitwise Operator/1, q/1, Mux2/1, Data Type Conversion/1, Logical Operator/2
  Logical Operator/1 -> Mux2/3, Mux/2, Data Type Conversion4/1, qtop/1
  carrier/1 -> PWM/2(carrier)
  Dead time/1 -> Data Type Conversion1/1
  Bitwise Operator/1 -> Logical Operator1/2, Mux1/2, Data Type Conversion3/1
  Dead time1/1 -> Data Type Conversion2/1
  Logical Operator1/1 -> Mux1/3, Mux/3, qbot/1, Data Type Conversion5/1
  Data Type Conversion1/1 -> Mux2/2, Logical Operator/1
  Data Type Conversion/1 -> Dead time/1
  Data Type Conversion2/1 -> Logical Operator1/1
  Data Type Conversion3/1 -> Dead time1/1
  Mux/1 -> qs/1
  Mux1/1 -> qbots/1
  Mux2/1 -> qtops/1
  Data Type Conversion4/1 -> q_top/1
  Data Type Conversion5/1 -> q_bot/1

== system a_CurrentController_IdealPWMVariousVbusFsw/Continuous Controller with PWM VBus=40, Fsw = 100 KHz/Switching Logic/Subsystem3 ==
  Carrier signal : simulink/Sources/Repeating Sequence  rep_seq_t=[0 .5 1]/fsw  rep_seq_y=[0 1 0]
  Scope : Scope
      settings: SaveName=ScopeData3
  Carrier : Outport
  wires:
  Carrier signal/1 -> Scope/1, Carrier/1

== system a_CurrentController_IdealPWMVariousVbusFsw/Continuous Controller with PWM VBus=200, Fsw = 100 KHz/Switching Logic/Leg 1/PWM ==
  d : Inport
  carrier : Inport  Port=2
  Relational Operator : RelationalOperator  OutDataTypeStr=boolean
  q : Outport
  wires:
  d/1 -> Relational Operator/1
  Relational Operator/1 -> q/1
  carrier/1 -> Relational Operator/2

== system a_CurrentController_IdealPWMVariousVbusFsw/Continuous Controller with PWM VBus=200, Fsw = 100 KHz/Switching Logic/Leg 2/PWM ==
  d : Inport
  carrier : Inport  Port=2
  Relational Operator : RelationalOperator  OutDataTypeStr=boolean
  q : Outport
  wires:
  d/1 -> Relational Operator/1
  Relational Operator/1 -> q/1
  carrier/1 -> Relational Operator/2

== system a_CurrentController_IdealPWMVariousVbusFsw/Continuous Controller with PWM VBus=40, Fsw = 100 KHz/Switching Logic/Leg 1/PWM ==
  d : Inport
  carrier : Inport  Port=2
  Relational Operator : RelationalOperator  OutDataTypeStr=boolean
  q : Outport
  wires:
  d/1 -> Relational Operator/1
  Relational Operator/1 -> q/1
  carrier/1 -> Relational Operator/2

== system a_CurrentController_IdealPWMVariousVbusFsw/Continuous Controller with PWM VBus=40, Fsw = 100 KHz/Switching Logic/Leg 2/PWM ==
  d : Inport
  carrier : Inport  Port=2
  Relational Operator : RelationalOperator  OutDataTypeStr=boolean
  q : Outport
  wires:
  d/1 -> Relational Operator/1
  Relational Operator/1 -> q/1
  carrier/1 -> Relational Operator/2
